simulink model "PIDController_1"  (Simulink 7.7)
settings: Solver=ode45  StartTime=0.0  StopTime=2  RelTol=1e-3
settings Model: Creator=Administrator  LastModifiedBy=Administrator
settings DebuggingCC: StrictBusMsg=Warning

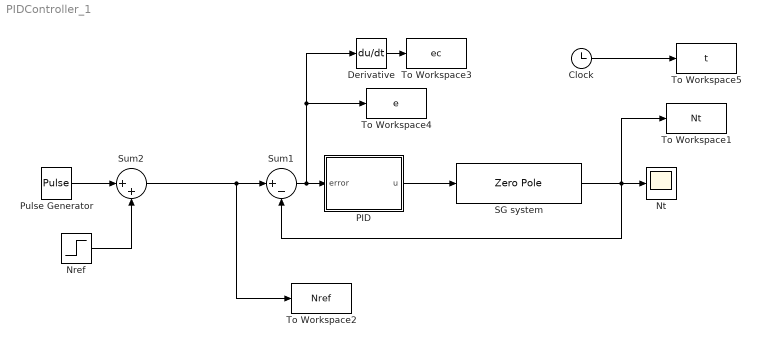
== system PIDController_1 ==
  Clock : Clock
      settings: Decimation=10
  Derivative : Derivative
  Nref : Step  Time=0  SampleTime=0
  Nt : Scope
      settings: TimeRange=3  YMin=0  YMax=2
  PID : Subsystem  mask{Kp=2.5, Ki=1.0, Kd=0}
      mask prompts: Kp "Proportional(Kp)"; Ki "Integral(Ki)"; Kd "Derivative(Kd)"
      mask help: Traditonal PID controller with three parameters:Proportional(Kp),Integral(Ki) and Derivative(Kd)
      mask Display: disp('PID Controller')
  Pulse Generator : DiscretePulseGenerator  PulseType=Time based  Amplitude=0.2  PhaseDelay=1
  SG system : ZeroPole  Zeros=[]  Poles=[-2.865 -40.235 ]  Gain=792
  Sum1 : Sum  Inputs=|+-
  Sum2 : Sum  Inputs=|++
  To Workspace1 : ToWorkspace  VariableName=Nt  SampleTime=0.001  SaveFormat=Array
  To Workspace2 : ToWorkspace  VariableName=Nref  SampleTime=0.001  SaveFormat=Array
  To Workspace3 : ToWorkspace  VariableName=ec  SampleTime=0.001  SaveFormat=Array
  To Workspace4 : ToWorkspace  VariableName=e  SampleTime=0.001  SaveFormat=Array
  To Workspace5 : ToWorkspace  VariableName=t  SampleTime=0.001  SaveFormat=Array
  wires:
  PID/1(u) -> SG system/1
  Sum1/1 -> PID/1(error), To Workspace4/1, Derivative/1
  SG system/1 -> Nt/1, Sum1/2, To Workspace1/1
  Derivative/1 -> To Workspace3/1
  Clock/1 -> To Workspace5/1
  Pulse Generator/1 -> Sum2/1
  Nref/1 -> Sum2/2
  Sum2/1 -> Sum1/1, To Workspace2/1

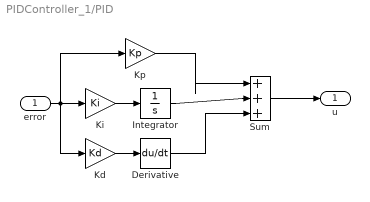
== system PIDController_1/PID ==
  error : Inport
  Derivative : Derivative
  Integrator : Integrator
  Kd : Gain  Gain=Kd
  Ki : Gain  Gain=Ki
  Kp : Gain  Gain=Kp
  Sum : Sum  Inputs=|+++
  u : Outport
  wires:
  error/1 -> Kp/1, Ki/1, Kd/1
  Ki/1 -> Integrator/1
  Kd/1 -> Derivative/1
  Kp/1 -> Sum/1
  Integrator/1 -> Sum/2
  Derivative/1 -> Sum/3
  Sum/1 -> u/1
